simulink model "sampleModel2023"  (R2023a)
settings: Solver=VariableStepAuto  StartTime=0.0  StopTime=10.0  RelTol=1e-3
libraries: hdlsllib x6, simulink x2
settings Model: Creator=user1  LastModifiedBy=user1

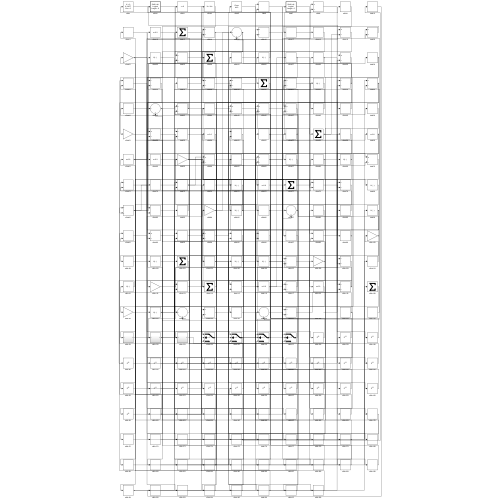
[thumbnail: Simulink's stored preview of the top-level diagram]
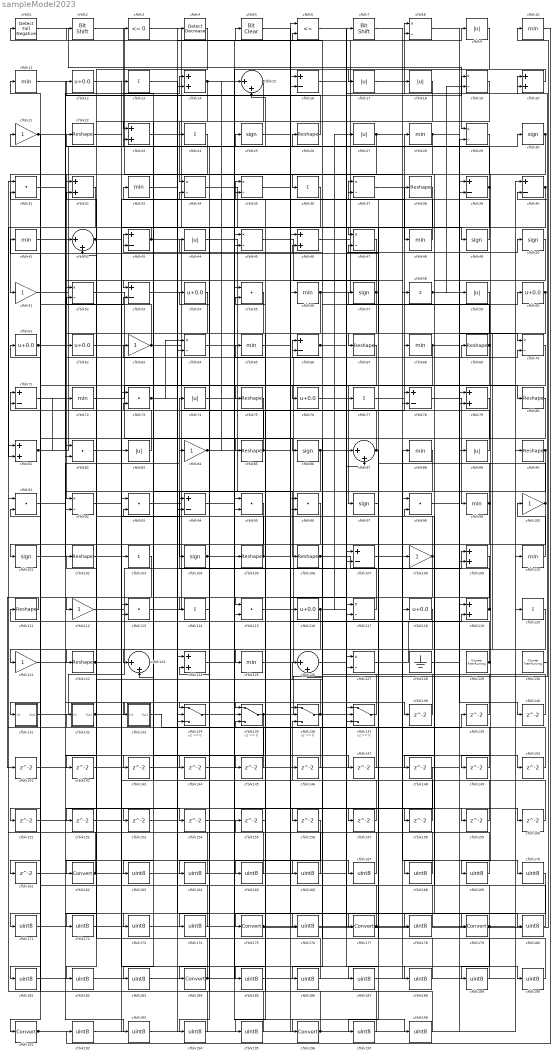
== system sampleModel2023 ==
  cfblk1 : hdlsllib/Logic and Bit Operations/Detect Fall Negative  vinit=0  OutDataTypeStr=boolean
  cfblk{10..11,28,33,41,48,56,65,68,72,88,99,110,125} (14 alike) : MinMax
  cfblk{21,51,63,84,100,108,112,121} (8 alike) : Gain
  cfblk{25,30,49..50,57,86,97,101,104} (9 alike) : Signum
  cfblk{22,26,38,67,69,75,80,85,90,102,105..106,111,122} (14 alike) : Reshape
  cfblk{13,24,36,58,77,103,114,120} (8 alike) : Sum  Inputs=+
  cfblk{16,39..40,43,53,66,71,78,94,107} (10 alike) : Sum  Inputs=+-
  cfblk{14,20,23,32,46,79,81,109,119,124} (10 alike) : Sum
  cfblk{31,55,73,82,91,93,95..96,98,113,115} (11 alike) : DotProduct  OutDataTypeStr=Inherit: Inherit via internal rule
  cfblk{12,54,60..62,76,116,118} (8 alike) : Bias  Bias=0.0  SaturateOnIntegerOverflow=off
  cfblk{8,19,29,34..35,37,45,47,52,64,70,92,117,127} (14 alike) : Product  Inputs=*/  RndMeth=Zero  SaturateOnIntegerOverflow=on
  cfblk{15,42,87,123,126} (5 alike) : Sum  Inputs=|++
  cfblk128 : Ground
  cfblk129 : hdlsllib/Sources/Counter Free-Running  NumBits=16  tsamp=-1
  cfblk130 : hdlsllib/Sources/Counter Free-Running  NumBits=16  tsamp=-1
  cfblk131 : Subsystem
      settings: LibrarySourceBlock=|
      | hdlsllib/Ports &
      | Subsystems/Subsystem
  cfblk132 : Subsystem
      settings: LibrarySourceBlock=|
      | hdlsllib/Ports &
      | Subsystems/Subsystem
  cfblk133 : Subsystem
      settings: LibrarySourceBlock=|
      | hdlsllib/Ports &
      | Subsystems/Subsystem
  cfblk{134..137} (4 alike) : Switch  SaturateOnIntegerOverflow=off  InputSameDT=off
  cfblk{138..161} (24 alike) : Delay  SampleTime=1
  cfblk{162,175,177,179,184,191,196} (7 alike) : DataTypeConversion  SaturateOnIntegerOverflow=off  RndMeth=Floor
  cfblk{163..174,176,178,180..183,185..190,192..195,197..198} (30 alike) : DataTypeConversion  OutDataTypeStr=uint8  SaturateOnIntegerOverflow=off  RndMeth=Floor
  cfblk{9,17..18,27,44,59,74,83,89} (9 alike) : Abs  SaturateOnIntegerOverflow=off
  cfblk2 : hdlsllib/Logic and Bit Operations/Bit Shift  mode=Shift Left Logical  N=0
  cfblk3 : hdlsllib/Logic and Bit Operations/Compare To Zero  relop=<=  OutDataTypeStr=boolean
  cfblk4 : simulink/Logic and Bit Operations/Detect Decrease  vinit=0.0  OutDataTypeStr=boolean
      settings: LibrarySourceBlock=|
      | hdlsllib/Logic and Bit
      | Operations/Detect
      | Decrease
  cfblk5 : simulink/Logic and Bit Operations/Bit Clear  iBit=0
      settings: LibrarySourceBlock=|
      | hdlsllib/Logic and Bit
      | Operations/Bit Clear
  cfblk6 : RelationalOperator  Operator=<=  OutDataTypeStr=boolean  InputSameDT=off
  cfblk7 : hdlsllib/Logic and Bit Operations/Bit Shift  mode=Shift Left Logical  N=0
  wires:
  cfblk54/1 -> cfblk92/1
  cfblk89/1 -> cfblk22/1
  cfblk113/1 -> cfblk66/1
  cfblk26/1 -> cfblk12/1
  cfblk99/1 -> cfblk71/2, cfblk182/1
  cfblk83/1 -> cfblk71/1
  cfblk109/1 -> cfblk111/1
  cfblk60/1 -> cfblk122/1, cfblk165/1
  cfblk110/1 -> cfblk100/1
  cfblk106/1 -> cfblk109/1, cfblk60/1
  cfblk68/1 -> cfblk70/1, cfblk171/1
  cfblk1/1 -> cfblk29/1
  cfblk4/1 -> cfblk162/1
  cfblk125/1 -> cfblk28/1
  cfblk52/1 -> cfblk76/1
  cfblk132/1(Out1) -> cfblk134/1, cfblk94/1
  cfblk8/1 -> cfblk109/2
  cfblk88/1 -> cfblk175/1
  cfblk135/1 -> cfblk20/1, cfblk119/2, cfblk163/1
  cfblk124/1 -> cfblk196/1
  cfblk117/1 -> cfblk74/1
  cfblk128/1 -> cfblk79/1
  cfblk2/1 -> cfblk36/1
  cfblk94/1 -> cfblk8/1
  cfblk74/1 -> cfblk106/1
  cfblk53/1 -> cfblk97/1
  cfblk137/1 -> cfblk43/1
  cfblk62/1 -> cfblk86/1
  cfblk98/1 -> cfblk39/1
  cfblk115/1 -> cfblk7/1
  cfblk49/1 -> cfblk33/1
  cfblk65/1 -> cfblk179/1
  cfblk29/1 -> cfblk92/2
  cfblk37/1 -> cfblk48/1
  cfblk70/1 -> cfblk115/1
  cfblk30/1 -> cfblk148/1, cfblk149/1
  cfblk81/1 -> cfblk3/1, cfblk53/2, cfblk72/1
  cfblk93/1 -> cfblk68/1
  cfblk75/1 -> cfblk85/1
  cfblk3/1 -> cfblk49/1
  cfblk67/1 -> cfblk121/1
  cfblk118/1 -> cfblk131/1(In1)
  cfblk19/1 -> cfblk34/1
  cfblk131/1(Out1) -> cfblk77/1
  cfblk27/1 -> cfblk51/1, cfblk150/1
  cfblk44/1 -> cfblk116/1
  cfblk77/1 -> cfblk78/1
  cfblk17/1 -> cfblk8/2
  cfblk123/1 -> cfblk93/2
  cfblk66/1 -> cfblk137/2, cfblk50/1
  cfblk112/1 -> cfblk16/1
  cfblk78/1 -> cfblk99/1
  cfblk48/1 -> cfblk26/1
  cfblk24/1 -> cfblk82/1
  cfblk43/1 -> cfblk75/1, cfblk42/1
  cfblk90/1 -> cfblk104/1, cfblk94/2
  cfblk119/1 -> cfblk112/1, cfblk37/2
  cfblk51/1 -> cfblk30/1
  cfblk34/1 -> cfblk136/2
  cfblk69/1 -> cfblk6/2, cfblk168/1
  cfblk108/1 -> cfblk13/1, cfblk114/1
  cfblk32/1 -> cfblk81/2
  cfblk102/1 -> cfblk177/1
  cfblk56/1 -> cfblk9/1, cfblk152/1
  cfblk130/1 -> cfblk40/2
  cfblk127/1 -> cfblk89/1
  cfblk42/1 -> cfblk47/1, cfblk142/1
  cfblk122/1 -> cfblk83/1, cfblk37/1
  cfblk72/1 -> cfblk80/1
  cfblk63/1 -> cfblk98/1, cfblk87/2, cfblk118/1, cfblk21/1, cfblk176/1
  cfblk5/1 -> cfblk56/1
  cfblk76/1 -> cfblk127/1
  cfblk87/1 -> cfblk35/1, cfblk187/1
  cfblk47/1 -> cfblk62/1
  cfblk101/1 -> cfblk84/1
  cfblk28/1 -> cfblk79/2, cfblk135/2
  cfblk85/1 -> cfblk63/1, cfblk52/2, cfblk38/1
  cfblk6/1 -> cfblk127/2
  cfblk40/1 -> cfblk52/1, cfblk174/1
  cfblk104/1 -> cfblk115/2, cfblk180/1
  cfblk61/1 -> cfblk14/1, cfblk25/1, cfblk70/2
  cfblk18/1 -> cfblk123/1
  cfblk45/1 -> cfblk78/2
  cfblk14/1 -> cfblk32/1, cfblk157/1
  cfblk15/1 -> cfblk23/1, cfblk24/1
  cfblk134/1 -> cfblk105/1
  cfblk9/1 -> cfblk45/2
  cfblk23/1 -> cfblk58/1
  cfblk46/1 -> cfblk18/1
  cfblk73/1 -> cfblk135/1, cfblk64/1
  cfblk64/1 -> cfblk119/1
  cfblk33/1 -> cfblk5/1
  cfblk103/1 -> cfblk191/1
  cfblk35/1 -> cfblk117/2
  cfblk116/1 -> cfblk69/1, cfblk27/1, cfblk151/1
  cfblk20/1 -> cfblk17/1
  cfblk96/1 -> cfblk125/1
  cfblk105/1 -> cfblk32/2, cfblk160/1
  cfblk100/1 -> cfblk41/1, cfblk153/1
  cfblk59/1 -> cfblk184/1
  cfblk58/1 -> cfblk19/2, cfblk140/1
  cfblk86/1 -> cfblk87/1, cfblk183/1
  cfblk129/1 -> cfblk34/2, cfblk169/1
  cfblk38/1 -> cfblk82/2
  cfblk84/1 -> cfblk35/2, cfblk15/1
  cfblk136/1 -> cfblk20/2, cfblk42/2
  cfblk114/1 -> cfblk44/1
  cfblk25/1 -> cfblk16/2
  cfblk39/1 -> cfblk67/1, cfblk23/2, cfblk15/2
  cfblk57/1 -> cfblk53/1, cfblk134/3
  cfblk21/1 -> cfblk101/1, cfblk19/1, cfblk96/2
  cfblk121/1 -> cfblk133/1(In1)
  cfblk92/1 -> cfblk138/1
  cfblk138/1 -> cfblk1/1
  cfblk133/1(Out1) -> cfblk139/1
  cfblk139/1 -> cfblk2/1
  cfblk140/1 -> cfblk66/2
  cfblk111/1 -> cfblk141/1
  cfblk141/1 -> cfblk136/1
  cfblk142/1 -> cfblk136/3
  cfblk71/1 -> cfblk143/1
  cfblk143/1 -> cfblk117/1
  cfblk12/1 -> cfblk144/1
  cfblk144/1 -> cfblk39/2
  cfblk13/1 -> cfblk145/1
  cfblk145/1 -> cfblk45/1
  cfblk146/1 -> cfblk73/2
  cfblk22/1 -> cfblk147/1
  cfblk147/1 -> cfblk81/1
  cfblk149/1 -> cfblk123/2
  cfblk150/1 -> cfblk47/2
  cfblk151/1 -> cfblk113/2
  cfblk153/1 -> cfblk14/2
  cfblk41/1 -> cfblk154/1
  cfblk155/1 -> cfblk135/3
  cfblk80/1 -> cfblk156/1
  cfblk157/1 -> cfblk46/2
  cfblk16/1 -> cfblk158/1
  cfblk158/1 -> cfblk93/1
  cfblk7/1 -> cfblk159/1
  cfblk159/1 -> cfblk137/1
  cfblk160/1 -> cfblk43/2
  cfblk79/1 -> cfblk161/1
  cfblk161/1 -> cfblk137/3
  cfblk162/1 -> cfblk64/2, cfblk61/1
  cfblk163/1 -> cfblk4/1
  cfblk55/1 -> cfblk164/1
  cfblk164/1 -> cfblk73/1
  cfblk165/1 -> cfblk55/1
  cfblk152/1 -> cfblk166/1
  cfblk166/1 -> cfblk55/2
  cfblk31/1 -> cfblk167/1
  cfblk167/1 -> cfblk146/1
  cfblk168/1 -> cfblk31/1
  cfblk169/1 -> cfblk31/2
  cfblk107/1 -> cfblk170/1
  cfblk171/1 -> cfblk107/1
  cfblk148/1 -> cfblk172/1
  cfblk172/1 -> cfblk107/2
  cfblk11/1 -> cfblk173/1
  cfblk173/1 -> cfblk6/1
  cfblk174/1 -> cfblk11/1
  cfblk175/1 -> cfblk10/1, cfblk40/1
  cfblk176/1 -> cfblk88/1
  cfblk177/1 -> cfblk96/1, cfblk90/1
  cfblk50/1 -> cfblk178/1
  cfblk178/1 -> cfblk102/1
  cfblk179/1 -> cfblk98/2, cfblk189/1
  cfblk180/1 -> cfblk65/1
  cfblk95/1 -> cfblk181/1
  cfblk181/1 -> cfblk108/1
  cfblk182/1 -> cfblk95/1
  cfblk183/1 -> cfblk95/2
  cfblk184/1 -> cfblk113/1, cfblk54/1
  cfblk170/1 -> cfblk185/1
  cfblk185/1 -> cfblk59/1
  cfblk120/1 -> cfblk186/1
  cfblk186/1 -> cfblk132/1(In1)
  cfblk187/1 -> cfblk120/1
  cfblk126/1 -> cfblk188/1
  cfblk188/1 -> cfblk57/1
  cfblk189/1 -> cfblk126/1
  cfblk82/1 -> cfblk190/1
  cfblk190/1 -> cfblk126/2
  cfblk191/1 -> cfblk134/2, cfblk29/2
  cfblk10/1 -> cfblk192/1
  cfblk192/1 -> cfblk103/1
  cfblk91/1 -> cfblk193/1
  cfblk193/1 -> cfblk46/1
  cfblk36/1 -> cfblk194/1
  cfblk194/1 -> cfblk91/1
  cfblk156/1 -> cfblk195/1
  cfblk195/1 -> cfblk91/2
  cfblk196/1 -> cfblk155/1, cfblk110/1
  cfblk97/1 -> cfblk197/1
  cfblk197/1 -> cfblk124/1
  cfblk154/1 -> cfblk198/1
  cfblk198/1 -> cfblk124/2

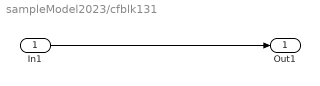
== system sampleModel2023/cfblk131 ==
  In1 : Inport
  Out1 : Outport
  wires:
  In1/1 -> Out1/1

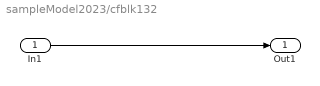
== system sampleModel2023/cfblk132 ==
  In1 : Inport
  Out1 : Outport
  wires:
  In1/1 -> Out1/1

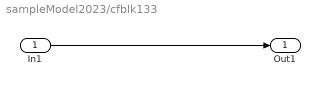
== system sampleModel2023/cfblk133 ==
  In1 : Inport
  Out1 : Outport
  wires:
  In1/1 -> Out1/1
